simulink model "ExperimentalLab3Assignments"  (R2020b)
settings: Solver=ode5  StartTime=0.0  StopTime=10  FixedStep=0.001  RelTol=1e-3
undefined symbols (not defined in the file): Aq, Bq, denH_w, DiscIntNeverNeededParam, enable_anti_windup, enable_integral_action, K, Kd, Ki, Kp, Kw, National_Instruments, Nu, numH_w, Nx, PCIe, sens, step_height, step_start_time, Tl, Ts
libraries: sldrtlib x12, simulink x8
settings Model: ExtModeTrigDuration=1000000  Creator=mustacchim  LastModifiedBy=mustacchim
settings RTWCC: Description=Simulink Desktop Real-Time  SystemTargetFile=sldrt.tlc  TemplateMakefile=sldrt.tmf  RTWCompilerOptimization=on
settings CodeAppCC: MaxIdLength=95
settings SimulinkDesktopRealTimeCC: TargetPreCompLibLocation=C:\Program Files\MATLAB\R2020b\toolbox\sldrt\lib\win64

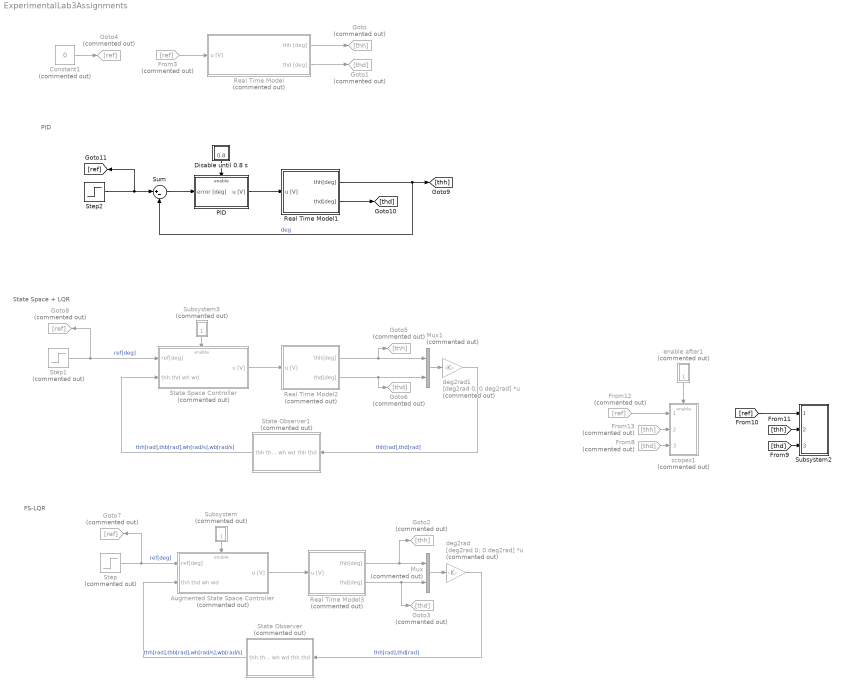
== system ExperimentalLab3Assignments ==
  note: FS-LQR
  note: PID
  note: State Space + LQR
  Augmented State Space Controller : Subsystem  Commented=on
  Constant1 : Constant  Commented=on  Value=0
  Disable until 0.8 s : Subsystem
  From12 : From  Commented=on  GotoTag=ref
  From13 : From  Commented=on  GotoTag=thh
  From3 : From  Commented=on  GotoTag=ref
  From8 : From  Commented=on  GotoTag=thd
  Goto : Goto  Commented=on  GotoTag=thh
  Goto1 : Goto  Commented=on  GotoTag=thd
  Goto2 : Goto  Commented=on  GotoTag=thh
  Goto3 : Goto  Commented=on  GotoTag=thd
  Goto4 : Goto  Commented=on  GotoTag=ref
  Goto5 : Goto  Commented=on  GotoTag=thh
  Goto6 : Goto  Commented=on  GotoTag=thd
  Goto7 : Goto  Commented=on  GotoTag=ref
  Goto8 : Goto  Commented=on  GotoTag=ref
  Mux : Mux  Commented=on  Inputs=2
  Mux1 : Mux  Commented=on  Inputs=2
  PID : Subsystem
  Real Time Model : Subsystem  Commented=on
  Real Time Model1 : Subsystem
  Real Time Model2 : Subsystem  Commented=on
  Real Time Model3 : Subsystem  Commented=on
  State Observer : Subsystem  Commented=on
  State Observer1 : Subsystem  Commented=on
  State Space Controller : Subsystem  Commented=on
  Step : Step  Commented=on  Time=step_start_time  After=step_height  SampleTime=0
  Step1 : Step  Commented=on  Time=step_start_time  After=step_height  SampleTime=0
  Step2 : Step  Time=step_start_time  After=step_height  SampleTime=0
  Subsystem : Subsystem  Commented=on
  Subsystem2 : Subsystem
  Subsystem3 : Subsystem  Commented=on
  Sum : Sum  Inputs=|+-
  deg2rad : Gain  Commented=on  Gain=[deg2rad 0; 0 deg2rad]  Multiplication=Matrix(K*u) (u vector)
  deg2rad1 : Gain  Commented=on  Gain=[deg2rad 0; 0 deg2rad]  Multiplication=Matrix(K*u) (u vector)
  enable after1 : Subsystem  Commented=on
  scopes1 : Subsystem  Commented=on
  wires:
  Real Time Model/2(thd [deg]) -> Goto1/1
  From3/1 -> Real Time Model/1(u [V])
  Constant1/1 -> Goto4/1
  Real Time Model/1(thh [deg]) -> Goto/1
  Subsystem3/1(0.8) -> State Space Controller/Enable
  Mux1/1 -> deg2rad1/1
  [ref] -> Subsystem2/1(ref[deg])
  [thh] -> Subsystem2/2(thh[deg])
  State Space Controller/1(u [V]) -> Real Time Model2/1(u [V])
  State Observer1/1(thh thd wh wd) -> State Space Controller/2(thh thd wh wd)  "thh[rad],thb[rad],wh[rad/s],wb[rad/s]"
  Real Time Model1/2(thd[deg]) -> [thd]
  PID/1(u [V]) -> Real Time Model1/1(u [V])
  Real Time Model1/1(thh[deg]) -> Sum/2, [thh]  "deg"
  Step1/1 -> State Space Controller/1(ref[deg]), Goto8/1  "ref[deg]"
  Mux/1 -> deg2rad/1
  Real Time Model2/1(thh[deg]) -> Goto5/1, Mux1/1
  deg2rad1/1 -> State Observer1/1(thh thd)  "thh[rad],thd[rad]"
  Real Time Model2/2(thd[deg]) -> Goto6/1, Mux1/2
  Step2/1 -> [ref], Sum/1
  enable after1/1(1.0 s) -> scopes1/Enable
  Real Time Model3/2(thd[deg]) -> Goto3/1, Mux/2
  From12/1 -> scopes1/1(ref[deg])
  From13/1 -> scopes1/2(thh[deg])
  State Observer/1(thh thd wh wd) -> Augmented State Space Controller/2(thh thd wh wd)  "thh[rad],thb[rad],wh[rad/s],wb[rad/s]"
  Sum/1 -> PID/1(error [deg])
  Step/1 -> Goto7/1, Augmented State Space Controller/1(ref[deg])  "ref[deg]"
  Disable until 0.8 s/1(0.8) -> PID/Enable
  From8/1 -> scopes1/3(thd[deg])
  Subsystem/1(0.8) -> Augmented State Space Controller/Enable
  Augmented State Space Controller/1(u [V]) -> Real Time Model3/1(u [V])
  [thd] -> Subsystem2/3(thd[deg])
  Real Time Model3/1(thh[deg]) -> Goto2/1, Mux/1
  deg2rad/1 -> State Observer/1(thh thd)  "thh[rad],thd[rad]"

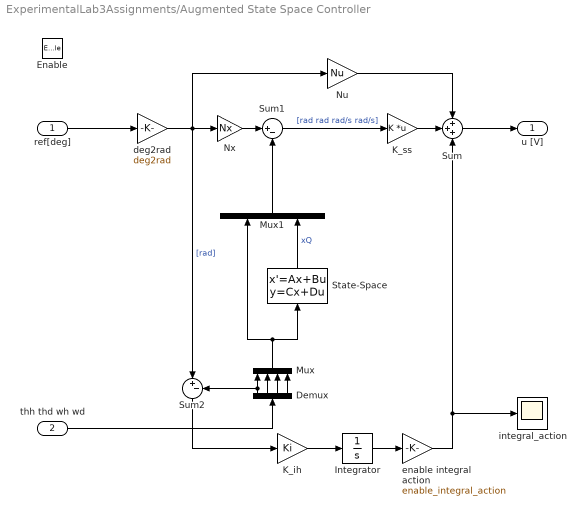
== system ExperimentalLab3Assignments/Augmented State Space Controller ==
  ref[deg] : Inport
  thh thd wh wd : Inport  Port=2
  Enable : EnablePort
  Demux : Demux
  Integrator : Integrator
  K_ih : Gain  Gain=Ki
  K_ss : Gain  Gain=K  Multiplication=Matrix(K*u) (u vector)
  Mux : Mux
  Mux1 : Mux  Inputs=2
  Nu : Gain  Gain=Nu
  Nx : Gain  Gain=Nx
  State-Space : StateSpace  A=Aq  B=Bq  C=eye(2,2)  D=zeros(2,4)  InitialCondition=0
  Sum : Sum  Inputs=+++
  Sum1 : Sum  Inputs=|+-
  Sum2 : Sum  Inputs=|+-
  deg2rad : Gain  Gain=deg2rad
  enable integral action : Gain  Gain=enable_integral_action
  integral_action : Scope
  u [V] : Outport
  wires:
  deg2rad/1 -> Nx/1, Nu/1, Sum2/1  "[rad]"
  K_ss/1 -> Sum/2
  Nx/1 -> Sum1/1
  ref[deg]/1 -> deg2rad/1
  Nu/1 -> Sum/1
  Sum/1 -> u [V]/1
  Sum1/1 -> K_ss/1  "[rad rad rad/s rad/s]"
  Demux/1 -> Mux/1, Sum2/2
  Demux/2 -> Mux/2
  Demux/3 -> Mux/3
  Demux/4 -> Mux/4
  thh thd wh wd/1 -> Demux/1
  Sum2/1 -> K_ih/1
  enable integral action/1 -> Sum/3, integral_action/1
  Mux/1 -> State-Space/1, Mux1/1
  State-Space/1 -> Mux1/2  "xQ"
  Mux1/1 -> Sum1/2
  K_ih/1 -> Integrator/1
  Integrator/1 -> enable integral action/1

== system ExperimentalLab3Assignments/Disable until 0.8 s ==
  Clock : Clock
  Interval Test : simulink/Logic and Bit Operations/Interval Test  IntervalClosedRight=on  uplimit=inf  IntervalClosedLeft=on  lowlimit=0.8  OutDataTypeStr=boolean
  0.8 : Outport
  wires:
  Clock/1 -> Interval Test/1
  Interval Test/1 -> 0.8/1

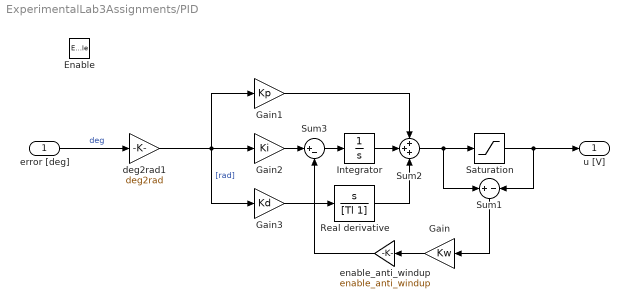
== system ExperimentalLab3Assignments/PID ==
  error [deg] : Inport
  Enable : EnablePort
  Gain : Gain  Gain=Kw
  Gain1 : Gain  Gain=Kp
  Gain2 : Gain  Gain=Ki
  Gain3 : Gain  Gain=Kd
  Integrator : Integrator
  Real derivative : TransferFcn  Numerator=[1 0]  Denominator=[Tl 1]
  Saturation : Saturate  UpperLimit=+10  LowerLimit=-10  LinearizeAsGain=off
  Sum1 : Sum  Inputs=+|-
  Sum2 : Sum  Inputs=+++
  Sum3 : Sum  Inputs=|+-
  deg2rad1 : Gain  Gain=deg2rad
  enable_anti_windup : Gain  Gain=enable_anti_windup
  u [V] : Outport
  wires:
  deg2rad1/1 -> Gain3/1, Gain1/1, Gain2/1  "[rad]"
  Gain1/1 -> Sum2/1
  error [deg]/1 -> deg2rad1/1  "deg"
  Gain2/1 -> Sum3/1
  Sum1/1 -> Gain/1
  Saturation/1 -> u [V]/1, Sum1/2
  Sum2/1 -> Sum1/1, Saturation/1
  Real derivative/1 -> Sum2/3
  Gain3/1 -> Real derivative/1
  Sum3/1 -> Integrator/1
  Integrator/1 -> Sum2/2
  Gain/1 -> enable_anti_windup/1
  enable_anti_windup/1 -> Sum3/2

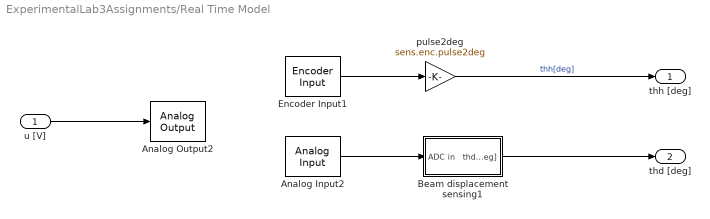
== system ExperimentalLab3Assignments/Real Time Model ==
  u [V] : Inport
  Analog Input2 : sldrtlib/Analog Input  SampleTime=0.001  MaxMissedTicks=10  ShowMissedTicks=off  YieldWhenWaiting=off  DrvName=National_Instruments/PCIe-6321  DrvAddress=4294967295  DrvOptions=[0 0 0 2 0 0 0]  Channels=[3,4]  RangeMode=1  VoltRange=2  DataType=1
      settings: AttributesFormatString=National Instruments\nPCIe-6321 [auto]
  Analog Output2 : sldrtlib/Analog Output  SampleTime=0.001  MaxMissedTicks=10  ShowMissedTicks=off  YieldWhenWaiting=off  DrvName=National_Instruments/PCIe-6321  DrvAddress=4294967295  DrvOptions=[0 0 0 2 0 0 0]  Channels=1  RangeMode=1  VoltRange=1  InitialValue=0  FinalValue=0
      settings: AttributesFormatString=National Instruments\nPCIe-6321 [auto]
  Beam displacement sensing1 : Subsystem
  Encoder Input1 : sldrtlib/Encoder Input  SampleTime=0.001  MaxMissedTicks=10  ShowMissedTicks=off  YieldWhenWaiting=off  DrvName=National_Instruments/PCIe-6321  DrvAddress=4294967295  DrvOptions=[0 0 0 2 0 0 0]  Channels=1  QuadMode=3  IndexPulse=2  InputFilter=Inf  DataType=1
      settings: AttributesFormatString=National Instruments\nPCIe-6321 [auto]
  pulse2deg : Gain  Gain=sens.enc.pulse2deg
  thh [deg] : Outport
  thd [deg] : Outport  Port=2
  wires:
  pulse2deg/1 -> thh [deg]/1  "thh[deg]"
  u [V]/1 -> Analog Output2/1
  Encoder Input1/1 -> pulse2deg/1
  Beam displacement sensing1/1(thd[deg]) -> thd [deg]/1
  Analog Input2/1 -> Beam displacement sensing1/1(ADC in)

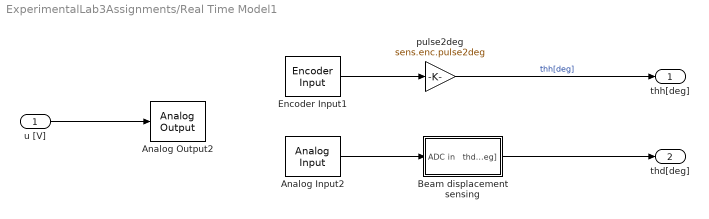
== system ExperimentalLab3Assignments/Real Time Model1 ==
  u [V] : Inport
  Analog Input2 : sldrtlib/Analog Input  SampleTime=0.001  MaxMissedTicks=10  ShowMissedTicks=off  YieldWhenWaiting=off  DrvName=National_Instruments/PCIe-6321  DrvAddress=4294967295  DrvOptions=[0 0 0 2 0 0 0]  Channels=[3,4]  RangeMode=1  VoltRange=2  DataType=1
      settings: AttributesFormatString=National Instruments\nPCIe-6321 [auto]
  Analog Output2 : sldrtlib/Analog Output  SampleTime=0.001  MaxMissedTicks=10  ShowMissedTicks=off  YieldWhenWaiting=off  DrvName=National_Instruments/PCIe-6321  DrvAddress=4294967295  DrvOptions=[0 0 0 2 0 0 0]  Channels=1  RangeMode=1  VoltRange=1  InitialValue=0  FinalValue=0
      settings: AttributesFormatString=National Instruments\nPCIe-6321 [auto]
  Beam displacement sensing : Subsystem
  Encoder Input1 : sldrtlib/Encoder Input  SampleTime=0.001  MaxMissedTicks=10  ShowMissedTicks=off  YieldWhenWaiting=off  DrvName=National_Instruments/PCIe-6321  DrvAddress=4294967295  DrvOptions=[0 0 0 2 0 0 0]  Channels=1  QuadMode=3  IndexPulse=2  InputFilter=Inf  DataType=1
      settings: AttributesFormatString=National Instruments\nPCIe-6321 [auto]
  pulse2deg : Gain  Gain=sens.enc.pulse2deg
  thh[deg] : Outport
  thd[deg] : Outport  Port=2
  wires:
  Encoder Input1/1 -> pulse2deg/1
  Beam displacement sensing/1(thd[deg]) -> thd[deg]/1
  Analog Input2/1 -> Beam displacement sensing/1(ADC in)
  pulse2deg/1 -> thh[deg]/1  "thh[deg]"
  u [V]/1 -> Analog Output2/1

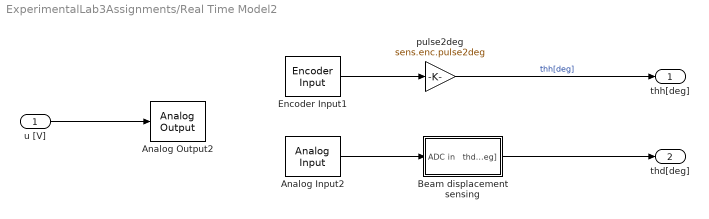
== system ExperimentalLab3Assignments/Real Time Model2 ==
  u [V] : Inport
  Analog Input2 : sldrtlib/Analog Input  SampleTime=0.001  MaxMissedTicks=10  ShowMissedTicks=off  YieldWhenWaiting=off  DrvName=National_Instruments/PCIe-6321  DrvAddress=4294967295  DrvOptions=[0 0 0 2 0 0 0]  Channels=[3,4]  RangeMode=1  VoltRange=2  DataType=1
      settings: AttributesFormatString=National Instruments\nPCIe-6321 [auto]
  Analog Output2 : sldrtlib/Analog Output  SampleTime=0.001  MaxMissedTicks=10  ShowMissedTicks=off  YieldWhenWaiting=off  DrvName=National_Instruments/PCIe-6321  DrvAddress=4294967295  DrvOptions=[0 0 0 2 0 0 0]  Channels=1  RangeMode=1  VoltRange=1  InitialValue=0  FinalValue=0
      settings: AttributesFormatString=National Instruments\nPCIe-6321 [auto]
  Beam displacement sensing : Subsystem
  Encoder Input1 : sldrtlib/Encoder Input  SampleTime=0.001  MaxMissedTicks=10  ShowMissedTicks=off  YieldWhenWaiting=off  DrvName=National_Instruments/PCIe-6321  DrvAddress=4294967295  DrvOptions=[0 0 0 2 0 0 0]  Channels=1  QuadMode=3  IndexPulse=2  InputFilter=Inf  DataType=1
      settings: AttributesFormatString=National Instruments\nPCIe-6321 [auto]
  pulse2deg : Gain  Gain=sens.enc.pulse2deg
  thh[deg] : Outport
  thd[deg] : Outport  Port=2
  wires:
  Encoder Input1/1 -> pulse2deg/1
  Beam displacement sensing/1(thd[deg]) -> thd[deg]/1
  Analog Input2/1 -> Beam displacement sensing/1(ADC in)
  pulse2deg/1 -> thh[deg]/1  "thh[deg]"
  u [V]/1 -> Analog Output2/1

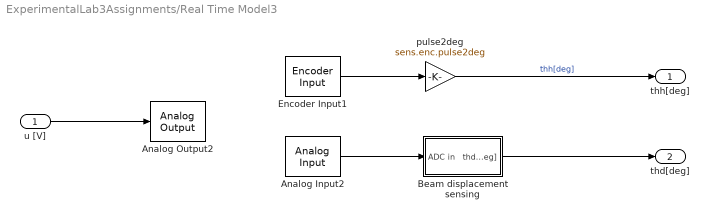
== system ExperimentalLab3Assignments/Real Time Model3 ==
  u [V] : Inport
  Analog Input2 : sldrtlib/Analog Input  SampleTime=0.001  MaxMissedTicks=10  ShowMissedTicks=off  YieldWhenWaiting=off  DrvName=National_Instruments/PCIe-6321  DrvAddress=4294967295  DrvOptions=[0 0 0 2 0 0 0]  Channels=[3,4]  RangeMode=1  VoltRange=2  DataType=1
      settings: AttributesFormatString=National Instruments\nPCIe-6321 [auto]
  Analog Output2 : sldrtlib/Analog Output  SampleTime=0.001  MaxMissedTicks=10  ShowMissedTicks=off  YieldWhenWaiting=off  DrvName=National_Instruments/PCIe-6321  DrvAddress=4294967295  DrvOptions=[0 0 0 2 0 0 0]  Channels=1  RangeMode=1  VoltRange=1  InitialValue=0  FinalValue=0
      settings: AttributesFormatString=National Instruments\nPCIe-6321 [auto]
  Beam displacement sensing : Subsystem
  Encoder Input1 : sldrtlib/Encoder Input  SampleTime=0.001  MaxMissedTicks=10  ShowMissedTicks=off  YieldWhenWaiting=off  DrvName=National_Instruments/PCIe-6321  DrvAddress=4294967295  DrvOptions=[0 0 0 2 0 0 0]  Channels=1  QuadMode=3  IndexPulse=2  InputFilter=Inf  DataType=1
      settings: AttributesFormatString=National Instruments\nPCIe-6321 [auto]
  pulse2deg : Gain  Gain=sens.enc.pulse2deg
  thh[deg] : Outport
  thd[deg] : Outport  Port=2
  wires:
  Encoder Input1/1 -> pulse2deg/1
  Beam displacement sensing/1(thd[deg]) -> thd[deg]/1
  Analog Input2/1 -> Beam displacement sensing/1(ADC in)
  pulse2deg/1 -> thh[deg]/1  "thh[deg]"
  u [V]/1 -> Analog Output2/1

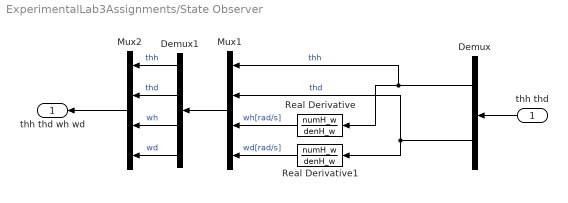
== system ExperimentalLab3Assignments/State Observer ==
  thh thd : Inport
  Demux : Demux  Outputs=2
  Demux1 : Demux
  Mux1 : Mux
  Mux2 : Mux
  Real Derivative : TransferFcn  Numerator=numH_w  Denominator=denH_w
  Real Derivative1 : TransferFcn  Numerator=numH_w  Denominator=denH_w
  thh thd wh wd : Outport
  wires:
  Real Derivative/1 -> Mux1/3  "wh[rad/s]"
  Demux/1 -> Real Derivative/1, Mux1/1  "thh"
  thh thd/1 -> Demux/1
  Real Derivative1/1 -> Mux1/4  "wd[rad/s]"
  Demux/2 -> Mux1/2, Real Derivative1/1  "thd"
  Mux2/1 -> thh thd wh wd/1
  Mux1/1 -> Demux1/1
  Demux1/1 -> Mux2/1  "thh"
  Demux1/2 -> Mux2/2  "thd"
  Demux1/3 -> Mux2/3  "wh"
  Demux1/4 -> Mux2/4  "wd"

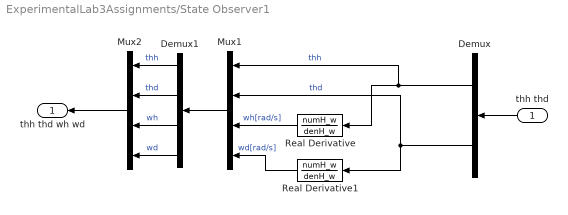
== system ExperimentalLab3Assignments/State Observer1 ==
  thh thd : Inport
  Demux : Demux  Outputs=2
  Demux1 : Demux
  Mux1 : Mux
  Mux2 : Mux
  Real Derivative : TransferFcn  Numerator=numH_w  Denominator=denH_w
  Real Derivative1 : TransferFcn  Numerator=numH_w  Denominator=denH_w
  thh thd wh wd : Outport
  wires:
  Real Derivative/1 -> Mux1/3  "wh[rad/s]"
  Demux/1 -> Real Derivative/1, Mux1/1  "thh"
  thh thd/1 -> Demux/1
  Real Derivative1/1 -> Mux1/4  "wd[rad/s]"
  Demux/2 -> Real Derivative1/1, Mux1/2  "thd"
  Mux2/1 -> thh thd wh wd/1
  Mux1/1 -> Demux1/1
  Demux1/1 -> Mux2/1  "thh"
  Demux1/2 -> Mux2/2  "thd"
  Demux1/3 -> Mux2/3  "wh"
  Demux1/4 -> Mux2/4  "wd"

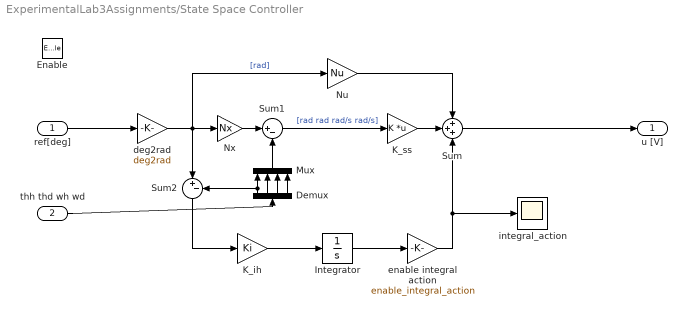
== system ExperimentalLab3Assignments/State Space Controller ==
  ref[deg] : Inport
  thh thd wh wd : Inport  Port=2
  Enable : EnablePort
  Demux : Demux
  Integrator : Integrator
  K_ih : Gain  Gain=Ki
  K_ss : Gain  Gain=K  Multiplication=Matrix(K*u) (u vector)
  Mux : Mux
  Nu : Gain  Gain=Nu
  Nx : Gain  Gain=Nx
  Sum : Sum  Inputs=+++
  Sum1 : Sum  Inputs=|+-
  Sum2 : Sum  Inputs=|+-
  deg2rad : Gain  Gain=deg2rad
  enable integral action : Gain  Gain=enable_integral_action
  integral_action : Scope
  u [V] : Outport
  wires:
  deg2rad/1 -> Nx/1, Nu/1, Sum2/1  "[rad]"
  K_ss/1 -> Sum/2
  Nx/1 -> Sum1/1
  ref[deg]/1 -> deg2rad/1
  Nu/1 -> Sum/1
  Sum/1 -> u [V]/1
  Sum1/1 -> K_ss/1  "[rad rad rad/s rad/s]"
  Demux/1 -> Mux/1, Sum2/2
  Demux/2 -> Mux/2
  Demux/3 -> Mux/3
  Demux/4 -> Mux/4
  thh thd wh wd/1 -> Demux/1
  Mux/1 -> Sum1/2
  Sum2/1 -> K_ih/1
  enable integral action/1 -> Sum/3, integral_action/1
  K_ih/1 -> Integrator/1
  Integrator/1 -> enable integral action/1

== system ExperimentalLab3Assignments/Subsystem ==
  Clock : Clock
  Interval Test : simulink/Logic and Bit Operations/Interval Test  IntervalClosedRight=on  uplimit=inf  IntervalClosedLeft=on  lowlimit=0.8  OutDataTypeStr=boolean
  0.8 : Outport
  wires:
  Clock/1 -> Interval Test/1
  Interval Test/1 -> 0.8/1

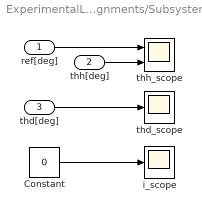
== system ExperimentalLab3Assignments/Subsystem2 ==
  ref[deg] : Inport
  thh[deg] : Inport  Port=2
  thd[deg] : Inport  Port=3
  Constant : Constant  Value=0
  i_scope : Scope
  thd_scope : Scope
  thh_scope : Scope  NumInputPorts=2
  wires:
  Constant/1 -> i_scope/1
  thd[deg]/1 -> thd_scope/1
  ref[deg]/1 -> thh_scope/1
  thh[deg]/1 -> thh_scope/2

== system ExperimentalLab3Assignments/Subsystem3 ==
  Clock : Clock
  Interval Test : simulink/Logic and Bit Operations/Interval Test  IntervalClosedRight=on  uplimit=inf  IntervalClosedLeft=on  lowlimit=0.8  OutDataTypeStr=boolean
  0.8 : Outport
  wires:
  Clock/1 -> Interval Test/1
  Interval Test/1 -> 0.8/1

== system ExperimentalLab3Assignments/enable after1 ==
  Clock : Clock
  Interval Test : simulink/Logic and Bit Operations/Interval Test  IntervalClosedRight=on  uplimit=inf  IntervalClosedLeft=on  lowlimit=1  OutDataTypeStr=boolean
  1.0 s : Outport
  wires:
  Interval Test/1 -> 1.0 s/1
  Clock/1 -> Interval Test/1

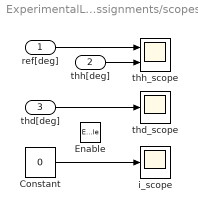
== system ExperimentalLab3Assignments/scopes1 ==
  ref[deg] : Inport
  thh[deg] : Inport  Port=2
  thd[deg] : Inport  Port=3
  Enable : EnablePort
  Constant : Constant  Value=0
  i_scope : Scope
  thd_scope : Scope
  thh_scope : Scope  NumInputPorts=2
  wires:
  thd[deg]/1 -> thd_scope/1
  Constant/1 -> i_scope/1
  thh[deg]/1 -> thh_scope/2
  ref[deg]/1 -> thh_scope/1

== system ExperimentalLab3Assignments/Real Time Model/Beam displacement sensing1 ==
  ADC in : Inport
  Bias Estimation : Subsystem
  Demux1 : Demux  Outputs=2
  Sum : Sum  Inputs=+-
  Sum1 : Sum  Inputs=+-|
  V2deg : Gain  Gain=sens.pot2.V2deg
  thd[deg] : Outport
  wires:
  Bias Estimation/1(thd_bias) -> Sum1/2
  Sum/1 -> V2deg/1
  Demux1/1 -> Sum/1  "vpot2"
  Demux1/2 -> Sum/2  "vref"
  Sum1/1 -> thd[deg]/1  "thd[deg]"
  V2deg/1 -> Sum1/1, Bias Estimation/1(thd)
  ADC in/1 -> Demux1/1

== system ExperimentalLab3Assignments/Real Time Model1/Beam displacement sensing ==
  ADC in : Inport
  Bias Estimation : Subsystem
  Demux1 : Demux  Outputs=2
  Sum : Sum  Inputs=+-
  Sum1 : Sum  Inputs=+-|
  V2deg : Gain  Gain=sens.pot2.V2deg
  thd[deg] : Outport
  wires:
  Bias Estimation/1(thd_bias) -> Sum1/2
  Sum/1 -> V2deg/1
  Demux1/1 -> Sum/1  "vpot2"
  Demux1/2 -> Sum/2  "vref"
  Sum1/1 -> thd[deg]/1  "thd[deg]"
  V2deg/1 -> Sum1/1, Bias Estimation/1(thd)
  ADC in/1 -> Demux1/1

== system ExperimentalLab3Assignments/Real Time Model2/Beam displacement sensing ==
  ADC in : Inport
  Bias Estimation : Subsystem
  Demux1 : Demux  Outputs=2
  Sum : Sum  Inputs=+-
  Sum1 : Sum  Inputs=+-|
  V2deg : Gain  Gain=sens.pot2.V2deg
  thd[deg] : Outport
  wires:
  Bias Estimation/1(thd_bias) -> Sum1/2
  Sum/1 -> V2deg/1
  Demux1/1 -> Sum/1  "vpot2"
  Demux1/2 -> Sum/2  "vref"
  Sum1/1 -> thd[deg]/1  "thd[deg]"
  V2deg/1 -> Sum1/1, Bias Estimation/1(thd)
  ADC in/1 -> Demux1/1

== system ExperimentalLab3Assignments/Real Time Model3/Beam displacement sensing ==
  ADC in : Inport
  Bias Estimation : Subsystem
  Demux1 : Demux  Outputs=2
  Sum : Sum  Inputs=+-
  Sum1 : Sum  Inputs=+-|
  V2deg : Gain  Gain=sens.pot2.V2deg
  thd[deg] : Outport
  wires:
  Bias Estimation/1(thd_bias) -> Sum1/2
  Sum/1 -> V2deg/1
  Demux1/1 -> Sum/1  "vpot2"
  Demux1/2 -> Sum/2  "vref"
  Sum1/1 -> thd[deg]/1  "thd[deg]"
  V2deg/1 -> Sum1/1, Bias Estimation/1(thd)
  ADC in/1 -> Demux1/1

== system ExperimentalLab3Assignments/Real Time Model/Beam displacement sensing1/Bias Estimation ==
  thd : Inport
  Average for 0.5 s : Subsystem
  Clock : Clock
  Gain : Gain  Gain=2
  Interval Test : simulink/Logic and Bit Operations/Interval Test  IntervalClosedRight=on  uplimit=0.7  IntervalClosedLeft=on  lowlimit=0.2  OutDataTypeStr=boolean
  thd_bias : Outport
  wires:
  Interval Test/1 -> Average for 0.5 s/Enable
  thd/1 -> Average for 0.5 s/1(In1)
  Clock/1 -> Interval Test/1
  Average for 0.5 s/1(Out1) -> Gain/1
  Gain/1 -> thd_bias/1

== system ExperimentalLab3Assignments/Real Time Model1/Beam displacement sensing/Bias Estimation ==
  thd : Inport
  Average for 0.5 s : Subsystem
  Clock : Clock
  Gain : Gain  Gain=2
  Interval Test : simulink/Logic and Bit Operations/Interval Test  IntervalClosedRight=on  uplimit=0.7  IntervalClosedLeft=on  lowlimit=0.2  OutDataTypeStr=boolean
  thd_bias : Outport
  wires:
  Interval Test/1 -> Average for 0.5 s/Enable
  thd/1 -> Average for 0.5 s/1(In1)
  Clock/1 -> Interval Test/1
  Average for 0.5 s/1(Out1) -> Gain/1
  Gain/1 -> thd_bias/1

== system ExperimentalLab3Assignments/Real Time Model2/Beam displacement sensing/Bias Estimation ==
  thd : Inport
  Average for 0.5 s : Subsystem
  Clock : Clock
  Gain : Gain  Gain=2
  Interval Test : simulink/Logic and Bit Operations/Interval Test  IntervalClosedRight=on  uplimit=0.7  IntervalClosedLeft=on  lowlimit=0.2  OutDataTypeStr=boolean
  thd_bias : Outport
  wires:
  Interval Test/1 -> Average for 0.5 s/Enable
  thd/1 -> Average for 0.5 s/1(In1)
  Clock/1 -> Interval Test/1
  Average for 0.5 s/1(Out1) -> Gain/1
  Gain/1 -> thd_bias/1

== system ExperimentalLab3Assignments/Real Time Model3/Beam displacement sensing/Bias Estimation ==
  thd : Inport
  Average for 0.5 s : Subsystem
  Clock : Clock
  Gain : Gain  Gain=2
  Interval Test : simulink/Logic and Bit Operations/Interval Test  IntervalClosedRight=on  uplimit=0.7  IntervalClosedLeft=on  lowlimit=0.2  OutDataTypeStr=boolean
  thd_bias : Outport
  wires:
  Interval Test/1 -> Average for 0.5 s/Enable
  thd/1 -> Average for 0.5 s/1(In1)
  Clock/1 -> Interval Test/1
  Average for 0.5 s/1(Out1) -> Gain/1
  Gain/1 -> thd_bias/1

== system ExperimentalLab3Assignments/Real Time Model/Beam displacement sensing1/Bias Estimation/Average for 0.5 s ==
  In1 : Inport
  Enable : EnablePort
  Discrete-Time Integrator : DiscreteIntegrator  SampleTime=Ts  ICPrevOutput=DiscIntNeverNeededParam  ICPrevScaledInput=DiscIntNeverNeededParam
  Out1 : Outport
  wires:
  In1/1 -> Discrete-Time Integrator/1
  Discrete-Time Integrator/1 -> Out1/1

== system ExperimentalLab3Assignments/Real Time Model1/Beam displacement sensing/Bias Estimation/Average for 0.5 s ==
  In1 : Inport
  Enable : EnablePort
  Discrete-Time Integrator : DiscreteIntegrator  SampleTime=Ts  ICPrevOutput=DiscIntNeverNeededParam  ICPrevScaledInput=DiscIntNeverNeededParam
  Out1 : Outport
  wires:
  In1/1 -> Discrete-Time Integrator/1
  Discrete-Time Integrator/1 -> Out1/1

== system ExperimentalLab3Assignments/Real Time Model2/Beam displacement sensing/Bias Estimation/Average for 0.5 s ==
  In1 : Inport
  Enable : EnablePort
  Discrete-Time Integrator : DiscreteIntegrator  SampleTime=Ts  ICPrevOutput=DiscIntNeverNeededParam  ICPrevScaledInput=DiscIntNeverNeededParam
  Out1 : Outport
  wires:
  In1/1 -> Discrete-Time Integrator/1
  Discrete-Time Integrator/1 -> Out1/1

== system ExperimentalLab3Assignments/Real Time Model3/Beam displacement sensing/Bias Estimation/Average for 0.5 s ==
  In1 : Inport
  Enable : EnablePort
  Discrete-Time Integrator : DiscreteIntegrator  SampleTime=Ts  ICPrevOutput=DiscIntNeverNeededParam  ICPrevScaledInput=DiscIntNeverNeededParam
  Out1 : Outport
  wires:
  In1/1 -> Discrete-Time Integrator/1
  Discrete-Time Integrator/1 -> Out1/1
